simulink model "unifiedModle_IR_MAYBE-2"  (R2023b)
settings: Solver=FixedStepAuto  StartTime=0.0  StopTime=inf  RelTol=1e-3  EnableMultiTasking=on
libraries: vexarmcortexlib x27, vexcommonlib x7, simulink x3
settings Model: Creator=carol  LastModifiedBy=ierdn
settings SolverCC: AutoInsertRateTranBlk=on
settings DataIOCC: LimitDataPoints=on  SignalLoggingSaveFormat=ModelDataLogs  ReturnWorkspaceOutputs=off
settings OptimizationCC: ExpressionDepthLimit=2147483647  LifeSpan=Inf  MaxStackSize=64  EfficientTunableParamExpr=on
settings DebuggingCC: MergeDetectMultiDrivingBlocksExec=none  InheritedTsInSrcMsg=none  FcnCallInpInsideContextMsg=warning  StateNameClashWarn=warning  SFUnexpectedBacktrackingDiag=warning  SFNoUnconditionalDefaultTransitionDiag=warning  SFExecutionAtInitializationDiag=none  ArithmeticOperatorsInVariantConditions=warning
settings HardwareCC: ProdBitPerPointer=32  ProdBitPerSizeT=32  ProdBitPerPtrDiffT=32  ProdLargestAtomicInteger=Long  ProdLargestAtomicFloat=Double  ProdIntDivRoundTo=Undefined  ProdWordSize=32  ProdHWDeviceType=ARM Compatible->ARM Cortex
settings ModelReferenceCC: EnableRefExpFcnMdlSchedulingChecks=on  PropagateSignalLabelsOutOfModel=off
settings SFSimCC: MATLABDynamicMemAlloc=off  CustomCodeUndefinedFunction=UseInterfaceOnly
settings RTWCC: Description=Embedded Coder  SystemTargetFile=ert.tlc  HardwareBoard=ARM Cortex-based VEX Microcontroller  TemplateMakefile=ert_default_tmf  Toolchain=GNU Tools for VEX ARM Cortex
settings CodeAppCC: IgnoreCustomStorageClasses=off  CustomSymbolStrType=$N$R$M  StateflowObjectComments=on  InternalIdentifier=Classic
settings ERTTargetCC: CodeReplacementLibrary=GCC ARM Cortex-M3  MultiwordLength=2048  ConvertIfToSwitch=off  SuppressUnreachableDefaultCases=off

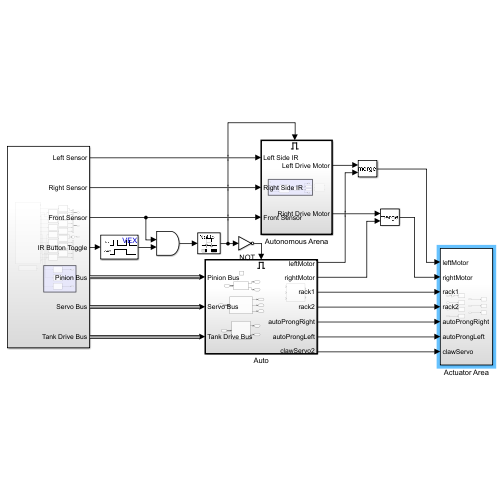
[thumbnail: Simulink's stored preview of the top-level diagram]
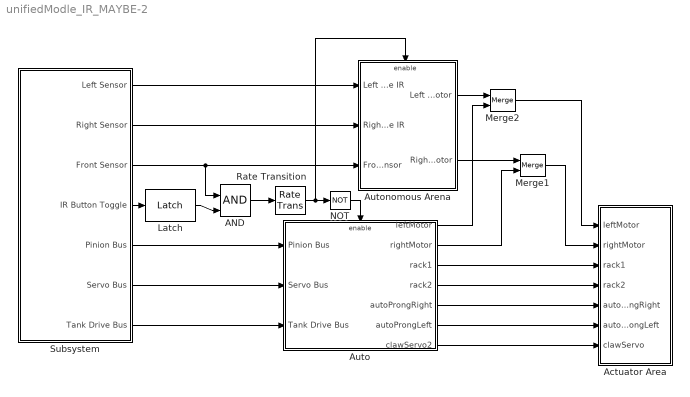
== system unifiedModle_IR_MAYBE-2 ==
  " NOT" : Logic  Operator=NOT  IconShape=distinctive  AllPortsSameDT=off  OutDataTypeStr=boolean
  AND : Logic  IconShape=distinctive  AllPortsSameDT=off  OutDataTypeStr=boolean
  Actuator Area : Subsystem
  Auto : Subsystem  TreatAsAtomicUnit=on
  Autonomous Arena : Subsystem  TreatAsAtomicUnit=on
  Latch : vexcommonlib/Latch  output0=off  BlockPlatform=vexarmcortex
  Merge1 : Merge
  Merge2 : Merge
  Rate Transition : RateTransition
  Subsystem : Subsystem
  wires:
  Auto/7(clawServo2) -> Actuator Area/7(clawServo)
  Auto/3(rack1) -> Actuator Area/3(rack1)
  Auto/5(autoProngRight) -> Actuator Area/5(autoProngRight)
  Auto/4(rack2) -> Actuator Area/4(rack2)
  Auto/6(autoProngLeft) -> Actuator Area/6(autoProngLeft)
  Auto/1(leftMotor) -> Merge2/2
  Auto/2(rightMotor) -> Merge1/2
  Merge1/1 -> Actuator Area/2(rightMotor)
  Merge2/1 -> Actuator Area/1(leftMotor)
  Autonomous Arena/1(Left Drive Motor) -> Merge2/1
  Autonomous Arena/2(Right Drive Motor) -> Merge1/1
  Subsystem/2(Right Sensor) -> Autonomous Arena/2(Right Side IR)
  Subsystem/3(Front Sensor) -> AND/1, Autonomous Arena/3(Front Sensor)
  Subsystem/1(Left Sensor) -> Autonomous Arena/1(Left Side IR)
  Subsystem/5(Pinion Bus) -> Auto/1(Pinion Bus)
  Subsystem/6(Servo Bus) -> Auto/2(Servo Bus)
  Subsystem/7(Tank Drive Bus) -> Auto/3(Tank Drive Bus)
  AND/1 -> Rate Transition/1
  Rate Transition/1 -> Autonomous Arena/Enable, " NOT"/1
  Subsystem/4(IR Button Toggle) -> Latch/1
  Latch/1 -> AND/2
  " NOT"/1 -> Auto/Enable

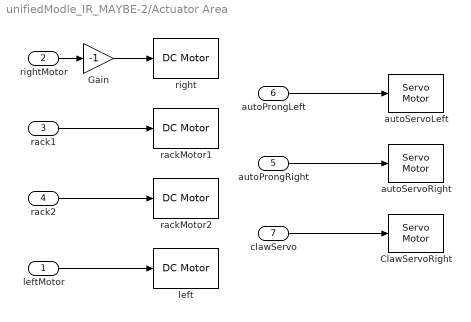
== system unifiedModle_IR_MAYBE-2/Actuator Area ==
  leftMotor : Inport
  rightMotor : Inport  Port=2
  rack1 : Inport  Port=3
  rack2 : Inport  Port=4
  autoProngRight : Inport  Port=5
  autoProngLeft : Inport  Port=6
  clawServo : Inport  Port=7
  ClawServoRight : vexarmcortexlib/Actuators/Servo Motor  motor=8  scaleFactor=60/127  SimulationOut=off
  Gain : Gain  Gain=-1
  autoServoLeft : vexarmcortexlib/Actuators/Servo Motor  motor=4  scaleFactor=60/127  SimulationOut=off
  autoServoRight : vexarmcortexlib/Actuators/Servo Motor  motor=7  scaleFactor=60/127  SimulationOut=off
  left : vexarmcortexlib/Actuators/DC Motor  motor=9  scaleFactor=1/13.5  SimulationOut=off
  rackMotor1 : vexarmcortexlib/Actuators/DC Motor  motor=6  scaleFactor=1/13.5  SimulationOut=off
  rackMotor2 : vexarmcortexlib/Actuators/DC Motor  motor=5  scaleFactor=1/13.5  SimulationOut=off
  right : vexarmcortexlib/Actuators/DC Motor  motor=2  scaleFactor=1/13.5  SimulationOut=off
  wires:
  leftMotor/1 -> left/1
  autoProngLeft/1 -> autoServoLeft/1
  rack1/1 -> rackMotor1/1
  rightMotor/1 -> Gain/1
  autoProngRight/1 -> autoServoRight/1
  clawServo/1 -> ClawServoRight/1
  rack2/1 -> rackMotor2/1
  Gain/1 -> right/1

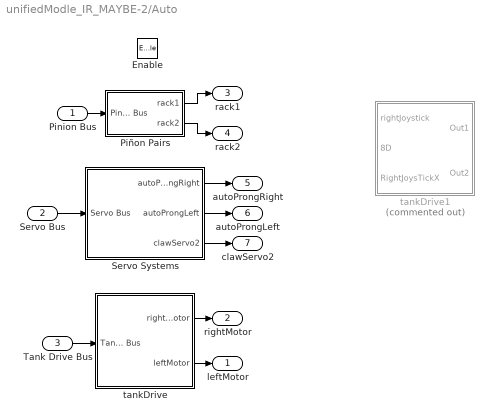
== system unifiedModle_IR_MAYBE-2/Auto ==
  Pinion Bus : Inport
  Servo Bus : Inport  Port=2
  Tank Drive Bus : Inport  Port=3
  Enable : EnablePort
  Piñon Pairs : Subsystem
  Servo Systems : Subsystem
  tankDrive : Subsystem
  tankDrive1 : Subsystem  Commented=on
  leftMotor : Outport
  rightMotor : Outport  Port=2
  rack1 : Outport  Port=3
  rack2 : Outport  Port=4
  autoProngRight : Outport  Port=5
  autoProngLeft : Outport  Port=6
  clawServo2 : Outport  Port=7
  wires:
  Servo Systems/1(autoProngRight) -> autoProngRight/1
  Servo Systems/3(clawServo2) -> clawServo2/1
  Servo Systems/2(autoProngLeft) -> autoProngLeft/1
  Piñon Pairs/1(rack1) -> rack1/1
  Servo Bus/1 -> Servo Systems/1(Servo Bus)
  Piñon Pairs/2(rack2) -> rack2/1
  Pinion Bus/1 -> Piñon Pairs/1(Pinion Bus)
  Tank Drive Bus/1 -> tankDrive/1(Tank Drive Bus)
  tankDrive/1(rightMotor) -> rightMotor/1
  tankDrive/2(leftMotor) -> leftMotor/1

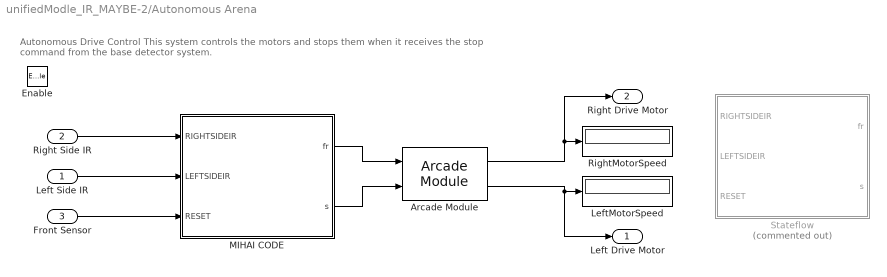
== system unifiedModle_IR_MAYBE-2/Autonomous Arena ==
  note: Autonomous Drive Control
      | This system controls the motors and stops them when it receives the stop command from the base detector system.
  Left Side IR : Inport
  Right Side IR : Inport  Port=2
  Front Sensor : Inport  Port=3
  Enable : EnablePort  StatesWhenEnabling=reset
  Arcade Module : vexcommonlib/Arcade Module  BlockPlatform=vexarmcortex
  LeftMotorSpeed : Display
  MIHAI CODE : Stateflow chart  TreatAsAtomicUnit=on
  RightMotorSpeed : Display
  Stateflow : Stateflow chart  Commented=on  TreatAsAtomicUnit=on
  Left Drive Motor : Outport
  Right Drive Motor : Outport  Port=2
  wires:
  Arcade Module/2 -> LeftMotorSpeed/1, Left Drive Motor/1
  Arcade Module/1 -> Right Drive Motor/1, RightMotorSpeed/1
  Front Sensor/1 -> MIHAI CODE/3(RESET)
  MIHAI CODE/1(fr) -> Arcade Module/1
  MIHAI CODE/2(s) -> Arcade Module/2
  Right Side IR/1 -> MIHAI CODE/1(RIGHTSIDEIR)
  Left Side IR/1 -> MIHAI CODE/2(LEFTSIDEIR)

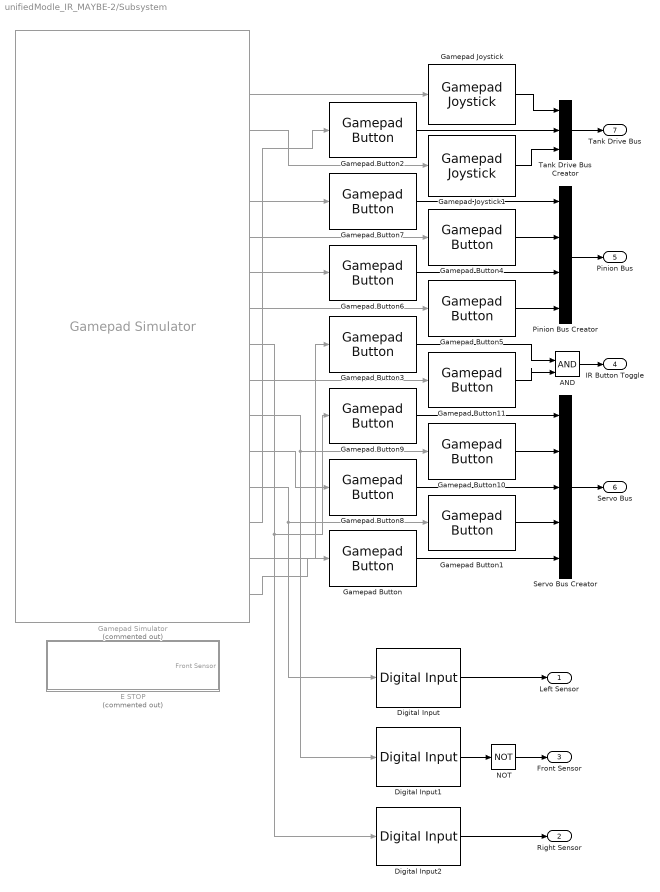
== system unifiedModle_IR_MAYBE-2/Subsystem ==
  AND : Logic  IconShape=distinctive  AllPortsSameDT=off  OutDataTypeStr=boolean
  Digital Input : vexarmcortexlib/Sensors/Digital Input  inChan=10  SimulationIn=on  SampleTime=0.02
  Digital Input1 : vexarmcortexlib/Sensors/Digital Input  inChan=11  SimulationIn=on  SampleTime=0.2
  Digital Input2 : vexarmcortexlib/Sensors/Digital Input  inChan=12  SimulationIn=on  SampleTime=0.02
  E STOP : Subsystem  Commented=on
  Gamepad Button : vexarmcortexlib/Gamepad/Gamepad Button  joystick=1  chan=7  button56=Up  button78=Left  SimulationIn=on  SampleTime=0.02
  Gamepad Button1 : vexarmcortexlib/Gamepad/Gamepad Button  joystick=1  chan=7  button56=Up  button78=Up  SimulationIn=on  SampleTime=0.02
  Gamepad Button10 : vexarmcortexlib/Gamepad/Gamepad Button  joystick=1  chan=8  button56=Up  button78=Right  SimulationIn=on  SampleTime=0.02
  Gamepad Button11 : vexarmcortexlib/Gamepad/Gamepad Button  joystick=1  chan=8  button56=Up  button78=Down  SimulationIn=on  SampleTime=0.02
  Gamepad Button2 : vexarmcortexlib/Gamepad/Gamepad Button  joystick=1  chan=7  button56=Up  button78=Right  SimulationIn=on  SampleTime=0.02
  Gamepad Button3 : vexarmcortexlib/Gamepad/Gamepad Button  joystick=1  chan=7  button56=Up  button78=Down  SimulationIn=on  SampleTime=0.02
  Gamepad Button4 : vexarmcortexlib/Gamepad/Gamepad Button  joystick=1  chan=5  button56=Down  button78=Down  SimulationIn=on  SampleTime=0.02
  Gamepad Button5 : vexarmcortexlib/Gamepad/Gamepad Button  joystick=1  chan=6  button56=Down  button78=Down  SimulationIn=on  SampleTime=0.02
  Gamepad Button6 : vexarmcortexlib/Gamepad/Gamepad Button  joystick=1  chan=6  button56=Up  button78=Down  SimulationIn=on  SampleTime=0.02
  Gamepad Button7 : vexarmcortexlib/Gamepad/Gamepad Button  joystick=1  chan=5  button56=Up  button78=Down  SimulationIn=on  SampleTime=0.02
  Gamepad Button8 : vexarmcortexlib/Gamepad/Gamepad Button  joystick=1  chan=8  button56=Up  button78=Left  SimulationIn=on  SampleTime=0.02
  Gamepad Button9 : vexarmcortexlib/Gamepad/Gamepad Button  joystick=1  chan=8  button56=Up  button78=Up  SimulationIn=on  SampleTime=0.02
  Gamepad Joystick : vexarmcortexlib/Gamepad/Gamepad Joystick  joystick=1  chan=2  SimulationIn=on  SampleTime=0.02
  Gamepad Joystick1 : vexarmcortexlib/Gamepad/Gamepad Joystick  joystick=1  chan=3  SimulationIn=on  SampleTime=0.02
  Gamepad Simulator : vexcommonlib/Gamepad Simulator  Commented=on  WhichPad=XBox Gamepad  JoyId=1  BlockPlatform=vexarmcortex
      settings: LibrarySourceBlock=vexarmcortexlib/Utilities/Gamepad Simulator
  NOT : Logic  Operator=NOT  Inputs=3  IconShape=distinctive  AllPortsSameDT=off  OutDataTypeStr=boolean
  Pinion Bus Creator : BusCreator  Inputs=4
  Servo Bus Creator : BusCreator  Inputs=5
  Tank Drive Bus Creator : BusCreator  Inputs=3
  Left Sensor : Outport
  Right Sensor : Outport  Port=2
  Front Sensor : Outport  Port=3
  IR Button Toggle : Outport  Port=4
  Pinion Bus : Outport  Port=5
  Servo Bus : Outport  Port=6
  Tank Drive Bus : Outport  Port=7
  wires:
  Gamepad Joystick1/1 -> Tank Drive Bus Creator/3
  Gamepad Simulator/12 -> Gamepad Button8/1
  Gamepad Simulator/8 -> Gamepad Button5/1
  Gamepad Joystick/1 -> Tank Drive Bus Creator/1
  Gamepad Simulator/7 -> Gamepad Button6/1
  Gamepad Button9/1 -> Servo Bus Creator/1
  Gamepad Button7/1 -> Pinion Bus Creator/1
  Gamepad Button10/1 -> Servo Bus Creator/2
  Gamepad Button2/1 -> Tank Drive Bus Creator/2
  Gamepad Simulator/11 -> Digital Input1/1, Gamepad Button10/1
  Gamepad Simulator/14 -> Gamepad Button2/1
  Gamepad Button6/1 -> Pinion Bus Creator/3
  Gamepad Button1/1 -> Servo Bus Creator/4
  Gamepad Simulator/5 -> Gamepad Button7/1
  Gamepad Button8/1 -> Servo Bus Creator/3
  Gamepad Simulator/2 -> Gamepad Joystick/1
  Gamepad Button11/1 -> AND/2
  Gamepad Button/1 -> Servo Bus Creator/5
  Gamepad Button5/1 -> Pinion Bus Creator/4
  Gamepad Simulator/13 -> Digital Input/1, Gamepad Button1/1
  Gamepad Button3/1 -> AND/1
  Gamepad Button4/1 -> Pinion Bus Creator/2
  Gamepad Simulator/6 -> Gamepad Button4/1
  Gamepad Simulator/9 -> Digital Input2/1, Gamepad Button9/1
  Gamepad Simulator/16 -> Gamepad Button/1
  Digital Input/1 -> Left Sensor/1
  Digital Input2/1 -> Right Sensor/1
  Digital Input1/1 -> NOT/1
  Gamepad Simulator/10 -> Gamepad Button11/1
  Gamepad Simulator/15 -> Gamepad Button3/1
  Gamepad Simulator/3 -> Gamepad Joystick1/1
  NOT/1 -> Front Sensor/1
  Pinion Bus Creator/1 -> Pinion Bus/1
  Servo Bus Creator/1 -> Servo Bus/1
  Tank Drive Bus Creator/1 -> Tank Drive Bus/1
  AND/1 -> IR Button Toggle/1

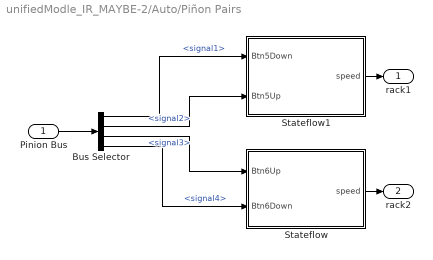
== system unifiedModle_IR_MAYBE-2/Auto/Piñon Pairs ==
  Pinion Bus : Inport
  Bus Selector : BusSelector  OutputSignals=signal1,signal2,signal3,signal4
  Stateflow : Stateflow chart  TreatAsAtomicUnit=on
  Stateflow1 : Stateflow chart  TreatAsAtomicUnit=on
  rack1 : Outport
  rack2 : Outport  Port=2
  wires:
  Stateflow/1(speed) -> rack2/1
  Stateflow1/1(speed) -> rack1/1
  Bus Selector/1 -> Stateflow1/1(Btn5Down)  "<signal1>"
  Pinion Bus/1 -> Bus Selector/1
  Bus Selector/2 -> Stateflow1/2(Btn5Up)  "<signal2>"
  Bus Selector/3 -> Stateflow/1(Btn6Up)  "<signal3>"
  Bus Selector/4 -> Stateflow/2(Btn6Down)  "<signal4>"

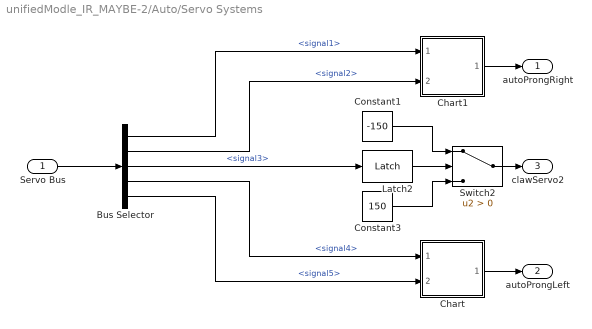
== system unifiedModle_IR_MAYBE-2/Auto/Servo Systems ==
  Servo Bus : Inport
  Bus Selector : BusSelector  OutputSignals=signal1,signal2,signal3,signal4,signal5
  Chart : Stateflow chart  TreatAsAtomicUnit=on
  Chart1 : Stateflow chart  TreatAsAtomicUnit=on
  Constant1 : Constant  Value=-150
  Constant3 : Constant  Value=150
  Latch2 : vexcommonlib/Latch  output0=off  BlockPlatform=vexarmcortex
      settings: LibrarySourceBlock=vexarmcortexlib/Utilities/Latch
  Switch2 : Switch  Criteria=u2 > Threshold  SaturateOnIntegerOverflow=off  InputSameDT=off
  autoProngRight : Outport
  autoProngLeft : Outport  Port=2
  clawServo2 : Outport  Port=3
  wires:
  Chart/1(angle) -> autoProngLeft/1
  Chart1/1(angle) -> autoProngRight/1
  Bus Selector/2 -> Chart1/2(Btn8Right)  "<signal2>"
  Servo Bus/1 -> Bus Selector/1
  Latch2/1 -> Switch2/2
  Constant1/1 -> Switch2/1
  Constant3/1 -> Switch2/3
  Switch2/1 -> clawServo2/1
  Bus Selector/1 -> Chart1/1(Btn8Up)  "<signal1>"
  Bus Selector/3 -> Latch2/1  "<signal3>"
  Bus Selector/4 -> Chart/1(Btn7Up)  "<signal4>"
  Bus Selector/5 -> Chart/2(Btn7Left)  "<signal5>"

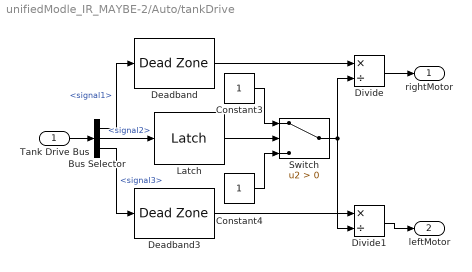
== system unifiedModle_IR_MAYBE-2/Auto/tankDrive ==
  Tank Drive Bus : Inport
  Bus Selector : BusSelector  OutputSignals=signal1,signal2,signal3
  Constant3 : Constant
  Constant4 : Constant
  Deadband : DeadZone  LowerValue=-9  UpperValue=9
  Deadband3 : DeadZone  LowerValue=-9  UpperValue=9
  Divide : Product  Inputs=*/
  Divide1 : Product  Inputs=*/
  Latch : vexcommonlib/Latch  output0=off  BlockPlatform=vexarmcortex
      settings: LibrarySourceBlock=vexarmcortexlib/Utilities/Latch
  Switch : Switch  Criteria=u2 > Threshold  SaturateOnIntegerOverflow=off  InputSameDT=off
  rightMotor : Outport
  leftMotor : Outport  Port=2
  wires:
  Constant4/1 -> Switch/3
  Constant3/1 -> Switch/1
  Divide1/1 -> leftMotor/1
  Latch/1 -> Switch/2
  Deadband3/1 -> Divide1/1
  Deadband/1 -> Divide/1
  Switch/1 -> Divide1/2, Divide/2
  Divide/1 -> rightMotor/1
  Tank Drive Bus/1 -> Bus Selector/1
  Bus Selector/2 -> Latch/1  "<signal2>"
  Bus Selector/1 -> Deadband/1  "<signal1>"
  Bus Selector/3 -> Deadband3/1  "<signal3>"

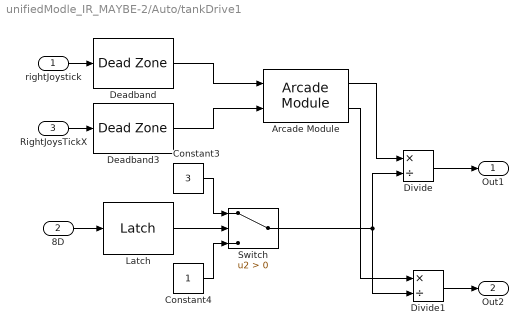
== system unifiedModle_IR_MAYBE-2/Auto/tankDrive1 ==
  rightJoystick : Inport
  "8D " : Inport  Port=2
  RightJoysTickX : Inport  Port=3
  Arcade Module : vexcommonlib/Arcade Module  BlockPlatform=vexarmcortex
  Constant3 : Constant  Value=3
  Constant4 : Constant
  Deadband : DeadZone  LowerValue=-9  UpperValue=9
  Deadband3 : DeadZone  LowerValue=-9  UpperValue=9
  Divide : Product  Inputs=*/
  Divide1 : Product  Inputs=*/
  Latch : vexcommonlib/Latch  output0=off  BlockPlatform=vexarmcortex
      settings: LibrarySourceBlock=vexarmcortexlib/Utilities/Latch
  Switch : Switch  Criteria=u2 > Threshold  SaturateOnIntegerOverflow=off  InputSameDT=off
  Out1 : Outport
  Out2 : Outport  Port=2
  wires:
  Constant4/1 -> Switch/3
  Constant3/1 -> Switch/1
  Latch/1 -> Switch/2
  Deadband/1 -> Arcade Module/1
  rightJoystick/1 -> Deadband/1
  Divide/1 -> Out1/1
  "8D "/1 -> Latch/1
  RightJoysTickX/1 -> Deadband3/1
  Divide1/1 -> Out2/1
  Arcade Module/2 -> Divide1/1
  Arcade Module/1 -> Divide/1
  Deadband3/1 -> Arcade Module/2
  Switch/1 -> Divide/2, Divide1/2

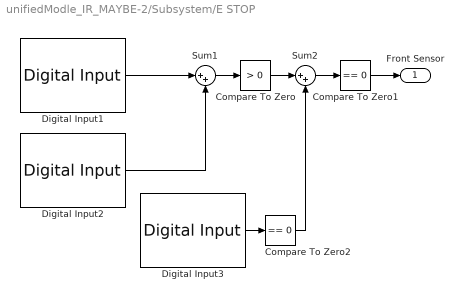
== system unifiedModle_IR_MAYBE-2/Subsystem/E STOP ==
  Compare To Zero : simulink/Logic and Bit Operations/Compare To Zero  relop=>  OutDataTypeStr=uint8
  Compare To Zero1 : simulink/Logic and Bit Operations/Compare To Zero  relop===  OutDataTypeStr=uint8
  Compare To Zero2 : simulink/Logic and Bit Operations/Compare To Zero  relop===  OutDataTypeStr=uint8
  Digital Input1 : vexarmcortexlib/Sensors/Digital Input  inChan=5  SimulationIn=off  SampleTime=0.2
  Digital Input2 : vexarmcortexlib/Sensors/Digital Input  inChan=6  SimulationIn=off  SampleTime=0.2
  Digital Input3 : vexarmcortexlib/Sensors/Digital Input  inChan=7  SimulationIn=off  SampleTime=0.2
  Sum1 : Sum  Inputs=|++
  Sum2 : Sum  Inputs=|++
  Front Sensor : Outport
  wires:
  Digital Input1/1 -> Sum1/1
  Sum1/1 -> Compare To Zero/1
  Digital Input2/1 -> Sum1/2
  Compare To Zero/1 -> Sum2/1
  Sum2/1 -> Compare To Zero1/1
  Compare To Zero1/1 -> Front Sensor/1
  Digital Input3/1 -> Compare To Zero2/1
  Compare To Zero2/1 -> Sum2/2

== stateflow chart unifiedModle_IR_MAYBE-2/Auto/Servo Systems/Chart ==
  state neutral
    angle=3;
  state buffer
    angle=3;
  state negative90
    angle=-40;
  state positive90
    angle=50;
  (default) -> neutral
  neutral -> negative90 [order 1] : [Btn7Left==1 && Btn7Up==0]
  neutral -> positive90 [order 2] : [Btn7Up==1 && Btn7Left==0]
  buffer -> neutral : [after(.75,sec)]
  negative90 -> buffer [order 1] : [Btn7Left==1 && Btn7Up==1]
  positive90 -> buffer [order 1] : [Btn7Up==1 && Btn7Left==1]
  negative90 -> positive90 [order 2] : [Btn7Left==0 && Btn7Up==1]
  positive90 -> negative90 [order 2] : [Btn7Up==0 && Btn7Left==1]
  data: Btn7Up input; Btn7Left input; angle output

== stateflow chart unifiedModle_IR_MAYBE-2/Auto/Piñon Pairs/Stateflow ==
  state rackIN
    entry:
    speed=-127;
  state STOPPED
    entry:
    speed=20;
  state rackOUT
    entry:
    speed=127;
  (default) -> STOPPED
  STOPPED -> rackOUT [order 2] : [Btn6Down==0 && Btn6Up==1]
  STOPPED -> rackIN [order 1] : [Btn6Down==1 && Btn6Up==0]
  rackIN -> STOPPED [order 1] : [Btn6Down==0]
  rackOUT -> STOPPED [order 1] : [Btn6Up==0]
  rackIN -> STOPPED [order 2] : [Btn6Down==1 && Btn6Up==1]
  rackOUT -> STOPPED [order 2] : [Btn6Down==1 && Btn6Up==1]
  data: Btn6Up input; Btn6Down input; speed output

== stateflow chart unifiedModle_IR_MAYBE-2/Auto/Piñon Pairs/Stateflow1 ==
  state rackIN
    entry:
    speed=-127;
  state STOPPED
    entry:
    speed=0;
  state rackOUT
    entry:
    speed=127;
  (default) -> STOPPED
  STOPPED -> rackOUT [order 2] : [Btn5Down==0 && Btn5Up==1]
  STOPPED -> rackIN [order 1] : [Btn5Down==1 && Btn5Up==0]
  rackIN -> STOPPED [order 1] : [Btn5Down==0]
  rackOUT -> STOPPED [order 1] : [Btn5Up==0]
  rackIN -> STOPPED [order 2] : [Btn5Down==1 && Btn5Up==1]
  rackOUT -> STOPPED [order 2] : [Btn5Down==1 && Btn5Up==1]
  data: speed output; Btn5Down input; Btn5Up input

== stateflow chart unifiedModle_IR_MAYBE-2/Autonomous Arena/Stateflow ==
  state STRAIGHT
    entry:
    fr = 127;
    s = 0;
  state GO_RIGHT
    entry:
    fr = 127;
    s = -100;
  state GO_LEFT
    entry:
    fr = 127;
    s = 100;
  state STOP
    entry:
    fr = 0;
    s = 0;
  (default) -> STRAIGHT
  GO_LEFT -> STRAIGHT [order 3] : [LEFTSIDEIR == 0 && RIGHTSIDEIR == 0]
  GO_RIGHT -> STRAIGHT [order 3] : [RIGHTSIDEIR == 0 && LEFTSIDEIR == 0]
  STRAIGHT -> GO_RIGHT [order 3] : [RIGHTSIDEIR == 0 && LEFTSIDEIR == 1]
  STRAIGHT -> GO_LEFT [order 2] : [LEFTSIDEIR == 0 && RIGHTSIDEIR ==1]
  STOP -> STRAIGHT [order 3] : [RIGHTSIDEIR == 0 && LEFTSIDEIR == 0 && RESET == 1]
  STRAIGHT -> STOP [order 1] : [RESET == 0]
  GO_LEFT -> GO_RIGHT [order 2] : [LEFTSIDEIR == 1 && RIGHTSIDEIR == 0]
  GO_RIGHT -> GO_LEFT [order 2] : [RIGHTSIDEIR == 1 && LEFTSIDEIR == 0]
  STOP -> GO_LEFT [order 2] : [RESET == 1 && LEFTSIDEIR == 0]
  GO_LEFT -> STOP [order 1] : [RESET == 0]
  STOP -> GO_RIGHT [order 1] : [RESET == 1 && RIGHTSIDEIR == 0]
  GO_RIGHT -> STOP [order 1] : [RESET == 0]
  data: RIGHTSIDEIR input; LEFTSIDEIR input; RESET input; fr output; s output

== stateflow chart unifiedModle_IR_MAYBE-2/Auto/Servo Systems/Chart1 ==
  state neutral
    angle=0;
  state buffer
    angle=0;
  state negative90
    angle=-30;
  state positive90
    angle=50;
  (default) -> neutral
  neutral -> negative90 [order 1] : [Btn8Right==1 && Btn8Up==0]
  neutral -> positive90 [order 2] : [Btn8Up==1 && Btn8Right==0]
  buffer -> neutral : [after(.75,sec)]
  positive90 -> buffer [order 1] : [Btn8Up==1 && Btn8Right==1]
  negative90 -> buffer [order 1] : [Btn8Right==1 && Btn8Up==1]
  negative90 -> positive90 [order 2] : [Btn8Right==0 && Btn8Up==1]
  positive90 -> negative90 [order 2] : [Btn8Up==0 && Btn8Right==1]
  data: angle output; Btn8Up input; Btn8Right input

== stateflow chart unifiedModle_IR_MAYBE-2/Autonomous Arena/MIHAI CODE ==
  state STRAIGHT
    entry:
    fr = 110;
    s = 0;
  state GO_RIGHT
    entry:
    fr = 90;
    s = -110;
  state GO_LEFT
    entry:
    fr = 90;
    s = 110;
  state STOP
    entry:
    fr = 0;
    s = 0;
  (default) -> STRAIGHT
  GO_LEFT -> STRAIGHT [order 3] : [LEFTSIDEIR == 0 && RIGHTSIDEIR == 0]
  GO_RIGHT -> STRAIGHT [order 3] : [RIGHTSIDEIR == 0 && LEFTSIDEIR == 0]
  STRAIGHT -> GO_RIGHT [order 3] : [RIGHTSIDEIR == 0 && LEFTSIDEIR == 1]
  STRAIGHT -> GO_LEFT [order 2] : [LEFTSIDEIR == 0 && RIGHTSIDEIR ==1]
  STOP -> STRAIGHT [order 3] : [RIGHTSIDEIR == 0 && LEFTSIDEIR == 0 && RESET == 1]
  STRAIGHT -> STOP [order 1] : [RESET == 0]
  GO_LEFT -> GO_RIGHT [order 2] : [LEFTSIDEIR == 1 && RIGHTSIDEIR == 0]
  GO_RIGHT -> GO_LEFT [order 2] : [RIGHTSIDEIR == 1 && LEFTSIDEIR == 0]
  STOP -> GO_LEFT [order 2] : [RESET == 1 && LEFTSIDEIR == 0]
  GO_LEFT -> STOP [order 1] : [RESET == 0]
  STOP -> GO_RIGHT [order 1] : [RESET == 1 && RIGHTSIDEIR == 0]
  GO_RIGHT -> STOP [order 1] : [RESET == 0]
  data: RIGHTSIDEIR input; LEFTSIDEIR input; RESET input; fr output; s output
